simulink model "PowertrainBestFuelController"  (R2019b)
settings: Solver=ode4  StartTime=0.0  StopTime=inf  FixedStep=.01  RelTol=1e-3  EnableMultiTasking=on
model workspace (MAT data in the model file):
  DCT_Param.Transmission.Ratios = [3.78 2.18 1.43 1.03 0.935 0.84]
  DCT_Param.Transmission.Shaft_Inertia_Odd = 0.0023
  DCT_Param.Transmission.Shaft_Inertia_Even = 0.0009
  DCT_Param.Transmission.Shaft_Inertia_Output = 0.008
  DCT_Param.Transmission.Gear_Inertia = 0.001
  DCT_Param.Transmission.Gear_Efficiency = 0.94
  DCT_Param.Transmission.Gear_Ang_Vel_Thr = 0.01
  DCT_Param.Transmission.Shaft_Velocity_Odd = 0
  DCT_Param.Transmission.Shaft_Velocity_Even = 0
  DCT_Param.Transmission.Shaft_Velocity_Output = 0
  DCT_Param.Transmission.Gear_Initial_Velocity = 0
  DCT_Param.Transmission.Abstract.Compliance = 100000
  DCT_Param.Transmission.Abstract.Damping = 10000
  DCT_Param.Transmission.Abstract.Ratio_Time_Const = 0.05
  DCT_Param.Transmission.Abstract.Shift_Gear_Delay = 25
  DCT_Param.Clutch.Torque_Radius = 130
  DCT_Param.Clutch.Num_Friction_Surfaces = 4
  DCT_Param.Clutch.Engagement_Piston_Area = 0.001
  DCT_Param.Clutch.Kinetic_Friction_Coeff = 0.3
  DCT_Param.Clutch.Static_Friction_Coeff = 0.31
  DCT_Param.Clutch.Derating_Factor = 1
  DCT_Param.Clutch.Clutch_Velocity_Tolerance = 0.001
  DCT_Param.Clutch.Threshold_Pressure = 1
  DCT_Param.Clutch.Drag_Torque_Coeff = 0
  DCT_Param.Dog_Clutch.Max_Torque = 1000
  DCT_Param.Dog_Clutch.Teeth_Mean_Radius = 50
  DCT_Param.Dog_Clutch.Tooth_Height = 10
  DCT_Param.Dog_Clutch.Ring_Hub_Clearance = 3
  DCT_Param.Dog_Clutch.Ring_Stop_Stiffness = 1000000
  DCT_Param.Dog_Clutch.Ring_Stop_Damping = 1000
  DCT_Param.Dog_Clutch.Shift_Linkage_Damping = 100
  DCT_Param.Dog_Clutch.Max_Engage_Velocity = 1000000
  DCT_Param.Dog_Clutch.Tooth_Engage_Overlap = 3
  DCT_Param.Vehicle.Mass = 1600
  DCT_Param.Vehicle.Wheels_Per_Axle = 2
  DCT_Param.Vehicle.Distance_CG_FrontAxle = 1.7
  DCT_Param.Vehicle.Distance_CG_RearAxle = 2
  DCT_Param.Vehicle.Distance_CG_Ground = 0.5
  DCT_Param.Vehicle.Frontal_Area = 3
  DCT_Param.Vehicle.Aero_Drag_Coeff = 0.4
  DCT_Param.Vehicle.Initial_Velocity = 0
  DCT_Param.Vehicle.Final_Drive_Ratio = 3.7
  DCT_Param.Vehicle.Final_Drive_Efficiency = 0.86
  DCT_Param.Vehicle.Final_Drive_Vel_Thresh = 0.01
  DCT_Param.Vehicle.Side_Shaft_Inertia = 0.01
  DCT_Param.Vehicle.Side_Shaft_Initial_Velocity = 0
  DCT_Param.Vehicle.Tire.Radius = 0.312
  DCT_Param.Vehicle.Tire.Inertia = 0.5
  DCT_Param.Vehicle.Tire.Initial_Velocity = 0
  DCT_Param.Vehicle.Tire.Slip_Vel_Thresh = 0.1
  DCT_Param.Vehicle.Tire.Nominal_Vertical_Load = 4000
  DCT_Param.Vehicle.Tire.C_Coeff = 1.685
  DCT_Param.Vehicle.Tire.D_Coeff = [1.21 -0.037]
  DCT_Param.Vehicle.Tire.E_Coeff = [0.344 0.095 -0.02 0]
  DCT_Param.Vehicle.Tire.BCD_Coeff = [21.51 -0.163 0.245]
  DCT_Param.Vehicle.Tire.H_Coeff = [-0.002 0.002]
  DCT_Param.Vehicle.Tire.V_Coeff = [0 0]
  DCT_Param.ICE.Max_Power = 100000
  DCT_Param.ICE.Speed_At_Max_Power = 5500
  DCT_Param.ICE.Max_Speed = 7000
  DCT_Param.ICE.Stall_Speed = 200
  DCT_Param.ICE.Shaft_Inertia = 0.2
  DCT_Param.ICE.Initial_Velocity = 800
  DCT_Param.ICE.Idle_Ref_Spd = 800
  DCT_Param.ICE.Engine_Time_Constant = 0.2
  DCT_Param.ICE.Initial_Normalized_Throttle = 0
  DCT_Param.ICE.Speed_Threshold = 20
  DCT_Param.ICE.FC.Speed_Vector = [0 368.421052632 736.842105263 1105.26315789 1473.68421053 1842.10526316 2210.52631579 2578.94736842 2947.36842105 3315.78947368 3684.21052632 4052.63157895 4421.05263158 4789.47368421 5157.89473684 5526.31578947 5894.73684211 6263.15789474 6631.57894737 7000]
  DCT_Param.ICE.FC.Torque_Vector = [0 10.5263157895 21.0526315789 31.5789473684 42.1052631579 52.6315789474 63.1578947368 73.6842105263 84.2105263158 94.7368421053 105.263157895 115.789473684 126.315789474 136.842105263 147.368421053 157.894736842 168.421052632 178.947368421 189.473684211 200]
  DCT_Param.ICE.FC.Consumption_Table = [0.262945178015 0.225304787522 0.201465019624 0.191425874321 0.195187351614 0.212749451502 0.244112173984 0.289275519063 0.348239486736 0.421004077004 0.507569289868 0.607935125326 ... (400 elements, 20x20)]
  DCT_Param.Shift_Map_Example.Pedal_Positions = [0.1 0.4 0.5 0.9]
  DCT_Param.Shift_Map_Example.Upshift_Speeds = [11  20  26  34.5  43; 14  26  35  44.5  55; 17  31  42  52.5  65; 21  39  52  66.5  80]
  DCT_Param.Shift_Map_Example.Downshift_Speeds = [8.9  17  23.6  32.4  40.8; 11.5  22.7  32  41.6  52.2; 14  27  38.1  50  62; 18  33  48  62.6  76.2]
  DCT_Param.Shift_Map_ORIG.Pedal_Positions = [0.1 0.4 0.5 0.9]
  DCT_Param.Shift_Map_ORIG.Upshift_Speeds = [11.5  23.5  35.5  45.5  55.5; 14.5  26.5  38.5  48.5  58.5; 17.5  29.5  41.5  51.5  61.5; 20.5  32.5  44.5  54.5  64.5]
  DCT_Param.Shift_Map_ORIG.Downshift_Speeds = [8.5  20.5  32.5  42.5  52.5; 11.5  23.5  35.5  45.5  55.5; 14.5  26.5  38.5  48.5  58.5; 17.5  29.5  41.5  51.5  61.5]
  DCT_Param.Shift_Map_OPT.Pedal_Positions = [0.1 0.4 0.5 0.9]
  DCT_Param.Shift_Map_OPT.Upshift_Speeds = [17.8469  29.8469  35.8159  41.2981  46.3004; 19.2469  33.9778  43.9778  53.9778  63.9778; 24.5469  41.9778  62.1778  78.5778  106.9778; 27.5469  59.3778  99.0445  109.0445  119.0445]
  DCT_Param.Shift_Map_OPT.Downshift_Speeds = [14.8469  26.8469  32.8159  38.2981  43.3004; 16.2469  30.9778  40.9778  50.9778  60.9778; 21.5469  38.9778  59.1778  75.5778  103.9778; 24.5469  56.3778  96.0445  106.0445  116.0445]
  DCT_Param.Shift_Map.Pedal_Positions = [0.1 0.4 0.5 0.9]
  DCT_Param.Shift_Map.Upshift_Speeds = [11.5  23.5  35.5  45.5  55.5; 14.5  26.5  38.5  48.5  58.5; 17.5  29.5  41.5  51.5  61.5; 20.5  32.5  44.5  54.5  64.5]
  DCT_Param.Shift_Map.Downshift_Speeds = [8.5  20.5  32.5  42.5  52.5; 11.5  23.5  35.5  45.5  55.5; 14.5  26.5  38.5  48.5  58.5; 17.5  29.5  41.5  51.5  61.5]
  DCT_Param.Control.Clutch.Min_Lock_Pressure = 2000000
  DCT_Param.Control.Clutch.Max_Lock_Pressure = 5000000
  DCT_Param.Control.Clutch.Max_Unlock_Pressure = 500000
  DCT_Param.Control.Engine_Start_RPM = 800
  DCT_Param.Control.Engine_Stop_RPM = 790
  DCT_Param.Control.Mode_Logic_TS = 0.1
  DCT_Param.Control.ICE.Kp = 0.02
  DCT_Param.Control.ICE.Ki = 0.01
  DCT_Param.Control.Gen.Kp = 10
  DCT_Param.Control.Gen.Ki = 3
  DCT_Param.Control.Mot.Kp = 500
  DCT_Param.Control.Mot.Ki = 300
  DCT_Param.Control.Veh_Spd.Kp = 0.02
  DCT_Param.Control.Veh_Spd.Ki = 0.04
  DCT_Param.Driver.Kp = 400
  DCT_Param.Driver.Ki = 0.001
  DCT_Param.Driver.Pedal_Filter_Const = 0.01
  DCT_Param.Dog_Clutches.Pulse_Delay = 50
  DCT_Param.Dog_Clutches.Pulse_Length = 20
  DCT_Param.Animation.Teeth_Ratios = [0.338461538462 0.555555555556 0.916666666667 0.96 1.17948717949 1.92307692308]
  DCT_Param.Animation.Teeth_Ratios_Reverse = [0.458333333333 0.75]
  DCT_Param.Shift_Map_OPT506.Pedal_Positions = [0.1 0.4 0.5 0.9]
  DCT_Param.Shift_Map_OPT506.Upshift_Speeds = [18  30.2  48.3  67.3322  77.3429; 20.1  36.85  66.6178  76.7537  86.7537; 21.1  40.25  71.0189  81.0189  91.7873; 24.1  63.75  80.7523  105.9489  115.9489]
  DCT_Param.Shift_Map_OPT506.Downshift_Speeds = [15  27.2  45.3  64.3322  74.3429; 17.1  33.85  63.6178  73.7537  83.7537; 18.1  37.25  68.0189  78.0189  88.7873; 21.1  60.75  77.7523  102.9489  112.9489]
  DCT_Param.Shift_Map_OPTAbsRea176.Pedal_Positions = [0.1 0.4 0.5 0.9]
  DCT_Param.Shift_Map_OPTAbsRea176.Upshift_Speeds = [17.8469  29.8469  35.7875  44.0901  49.4243; 18.9219  34.1312  45.8256  59.7585  69.7585; 32.1719  43.4585  53.51  103.2151  114.6401; 35.1719  59.2585  99.5217  109.5217  119.5217]
  DCT_Param.Shift_Map_OPTAbsRea176.Downshift_Speeds = [14.8469  26.8469  32.7875  41.0901  46.4243; 15.9219  31.1312  42.8256  56.7585  66.7585; 29.1719  40.4585  50.51  100.2151  111.6401; 32.1719  56.2585  96.5217  106.5217  116.5217]
  Downshift_Speeds = [9.5625  23.0625  36.5625  47.8125  59.0625  68.90625  78.75; 12.9375  26.4375  39.9375  51.1875  62.4375  72.84375  83.25; 16.3125  29.8125  43.3125  54.5625  65.8125  76.78125  87.75; 19.6875  33.1875  46.6875  57.9375  69.1875  80.71875  92.25]
  Pedal_Positions = [0.1 0.4 0.5 0.9]
  Upshift_Speeds = [12.9375  26.4375  39.9375  51.1875  62.4375  72.84375  83.25; 16.3125  29.8125  43.3125  54.5625  65.8125  76.78125  87.75; 19.6875  33.1875  46.6875  57.9375  69.1875  80.71875  92.25; 33  52.5  77.25  100.5  138.75  161.875  185]
settings Model: ModifiedByFormat=The MathWorks, Inc.  Creator=The MathWorks, Inc.  LastModifiedBy=The MathWorks, Inc.
settings DataIOCC: SaveFormat=StructureWithTime  DSMLogging=off  ReturnWorkspaceOutputs=off
settings DebuggingCC: ArithmeticOperatorsInVariantConditions=warning
settings SFSimCC: SimUseLocalCustomCode=off  CustomCodeUndefinedFunction=UseInterfaceOnly
settings RTWCC: RTWUseLocalCustomCode=off
settings CodeAppCC: StateflowObjectComments=on
settings GRTTargetCC: TargetLangStandard=C89/C90 (ANSI)
settings ConfigComp: CovMetricSettings=dsw  CovHtmlReporting=on  CovSaveCumulativeToWorkspaceVar=on  CovSaveSingleToWorkspaceVar=on  CovShowResultsExplorer=off  CovExternalEMLEnable=off

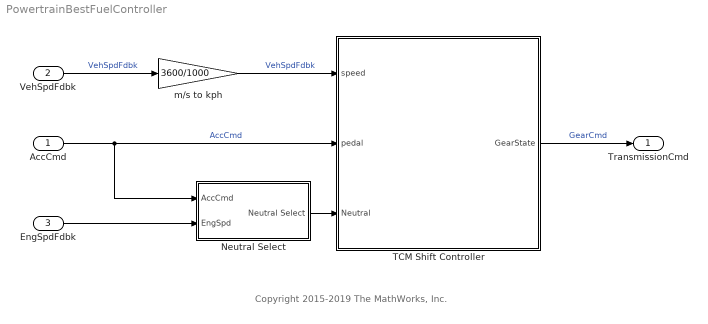
== system PowertrainBestFuelController ==
  note: Copyright 2015-2019 The MathWorks, Inc.
  AccCmd : Inport
  VehSpdFdbk : Inport  Port=2
  EngSpdFdbk : Inport  Port=3
  Neutral Select : Subsystem
  TCM Shift Controller : Stateflow chart  TreatAsAtomicUnit=on
  m/s to kph : Gain  Gain=3600/1000
  TransmissionCmd : Outport  VectorParamsAs1DForOutWhenUnconnected=off
  wires:
  AccCmd/1 -> Neutral Select/1(AccCmd), TCM Shift Controller/2(pedal)  "AccCmd"
  m/s to kph/1 -> TCM Shift Controller/1(speed)  "VehSpdFdbk"
  VehSpdFdbk/1 -> m/s to kph/1  "VehSpdFdbk"
  EngSpdFdbk/1 -> Neutral Select/2(EngSpd)
  Neutral Select/1(Neutral Select) -> TCM Shift Controller/3(Neutral)
  TCM Shift Controller/1(GearState) -> TransmissionCmd/1  "GearCmd"

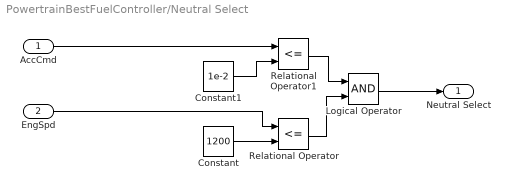
== system PowertrainBestFuelController/Neutral Select ==
  AccCmd : Inport
  EngSpd : Inport  Port=2
  Constant : Constant  Value=1200
  Constant1 : Constant  Value=1e-2
  Logical Operator : Logic  AllPortsSameDT=off  OutDataTypeStr=boolean
  Relational Operator : RelationalOperator  Operator=<=  OutDataTypeStr=boolean  RndMeth=Simplest
  Relational Operator1 : RelationalOperator  Operator=<=  OutDataTypeStr=boolean  RndMeth=Simplest
  Neutral Select : Outport  VectorParamsAs1DForOutWhenUnconnected=off
  wires:
  EngSpd/1 -> Relational Operator/1
  Relational Operator1/1 -> Logical Operator/1
  AccCmd/1 -> Relational Operator1/1
  Constant1/1 -> Relational Operator1/2
  Logical Operator/1 -> Neutral Select/1
  Constant/1 -> Relational Operator/2
  Relational Operator/1 -> Logical Operator/2

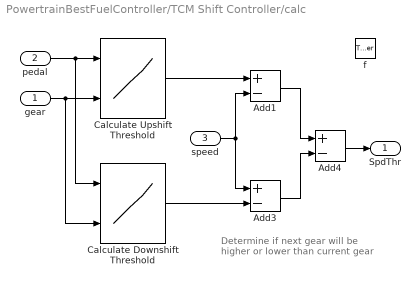
== system PowertrainBestFuelController/TCM Shift Controller/calc ==
  note: Determine if next gear will be
      | higher or lower than current gear
  gear : Inport
  pedal : Inport  Port=2
  speed : Inport  Port=3
  f : TriggerPort  TriggerType=function-call  VariantControl=Variant  StatesWhenEnabling=reset
      settings: CopyFcn=Stateflow.SLINSF.SimulinkMan.removeBlockPreDeleteFcn  PreDeleteFcn=Stateflow.SLINSF.SimulinkMan.unsafePredeleteFcn
  Add1 : Sum  Inputs=+-
  Add3 : Sum  Inputs=+-
  Add4 : Sum  Inputs=+-
  Calculate Upshift Threshold : Lookup_n-D  BreakpointsForDimension1=Pedal_Positions  BreakpointsForDimension2=1:7  Table=Upshift_Speeds  ExtrapMethod=Clip  UseLastTableValue=on  InternalRulePriority=Speed  RndMeth=Simplest  InputSameDT=on
  Calculate Downshift Threshold : Lookup_n-D  BreakpointsForDimension1=Pedal_Positions  BreakpointsForDimension2=2:8  Table=Downshift_Speeds  ExtrapMethod=Clip  UseLastTableValue=on  InternalRulePriority=Speed  RndMeth=Simplest  InputSameDT=on
  SpdThr : Outport  VectorParamsAs1DForOutWhenUnconnected=off
  wires:
  pedal/1 -> Calculate Downshift Threshold/1, Calculate Upshift Threshold/1
  gear/1 -> Calculate Downshift Threshold/2, Calculate Upshift Threshold/2
  Calculate Downshift Threshold/1 -> Add3/2
  Calculate Upshift Threshold/1 -> Add1/1
  speed/1 -> Add1/2, Add3/1
  Add1/1 -> Add4/1
  Add3/1 -> Add4/2
  Add4/1 -> SpdThr/1

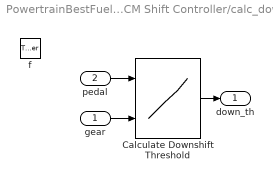
== system PowertrainBestFuelController/TCM Shift Controller/calc_down ==
  gear : Inport
  pedal : Inport  Port=2
  f : TriggerPort  TriggerType=function-call  VariantControl=Variant  StatesWhenEnabling=reset
      settings: CopyFcn=Stateflow.SLINSF.SimulinkMan.removeBlockPreDeleteFcn  PreDeleteFcn=Stateflow.SLINSF.SimulinkMan.unsafePredeleteFcn
  Calculate Downshift Threshold : Lookup_n-D  BreakpointsForDimension1=Pedal_Positions  BreakpointsForDimension2=2:8  Table=Downshift_Speeds  ExtrapMethod=Clip  UseLastTableValue=on  InternalRulePriority=Speed  RndMeth=Simplest  InputSameDT=on
  down_th : Outport  VectorParamsAs1DForOutWhenUnconnected=off
  wires:
  Calculate Downshift Threshold/1 -> down_th/1
  gear/1 -> Calculate Downshift Threshold/2
  pedal/1 -> Calculate Downshift Threshold/1

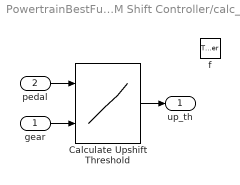
== system PowertrainBestFuelController/TCM Shift Controller/calc_up ==
  gear : Inport
  pedal : Inport  Port=2
  f : TriggerPort  TriggerType=function-call  VariantControl=Variant  StatesWhenEnabling=reset
      settings: CopyFcn=Stateflow.SLINSF.SimulinkMan.removeBlockPreDeleteFcn  PreDeleteFcn=Stateflow.SLINSF.SimulinkMan.unsafePredeleteFcn
  Calculate Upshift Threshold : Lookup_n-D  BreakpointsForDimension1=Pedal_Positions  BreakpointsForDimension2=1:7  Table=Upshift_Speeds  ExtrapMethod=Clip  UseLastTableValue=on  InternalRulePriority=Speed  RndMeth=Simplest  InputSameDT=on
  up_th : Outport  VectorParamsAs1DForOutWhenUnconnected=off
  wires:
  Calculate Upshift Threshold/1 -> up_th/1
  pedal/1 -> Calculate Upshift Threshold/1
  gear/1 -> Calculate Upshift Threshold/2

== stateflow chart PowertrainBestFuelController/TCM Shift Controller ==
  settings: sampleTime=0.01
  state GearState [parallel]
    settings: executionOrder=1
    state Neutral
      en:
      GearState = 0;
    state G1
      en:
      GearState = 1;
    state G2
      en:
      GearState = 2;
      du:
      [SpdThr] = calc(2,pedal,speed);
    state G3
      en:
      GearState = 3;
      du:
      [SpdThr] = calc(3,pedal,speed);
    state G8
      en:
      GearState = 8;
    state G7
      en:
      GearState = 7;
    state G6
      en:
      GearState = 6;
    state G5
      en:GearState=5;
      du:[SpdThr]=calc(5,pedal,speed);
    state G4
      en:
      GearState = 4;
      du:
      [SpdThr] = calc(4,pedal,speed);
    (default) -> G1
    Neutral -> G1 : [~Neutral]
    G1 -> G2 [order 1] : Up
    G2 -> G3 [order 1] : Up
    G1 -> Neutral [order 2] : [Neutral]
    G2 -> G1 [order 2] : Down
    G3 -> G2 [order 2] : Down
    G3 -> G4 [order 1] : Up
    G4 -> G3 [order 2] : Down
    G7 -> G8 [order 1] : Up
    G5 -> G6 [order 1] : Up
    G6 -> G7 [order 1] : Up
    G4 -> G5 [order 1] : Up
    G5 -> G4 [order 2] : Down
    G6 -> G5 [order 2] : Down
    G7 -> G6 [order 2] : Down
    G8 -> G7 : Down
  state SelectionState [parallel]
    du:[up_th]=calc_up(GearState,pedal);
    du:[down_th]=calc_down(GearState,pedal);
    settings: executionOrder=2
    state SteadyState
      en:
      clutchControl = 0;
    state preDownShifting
    state preUpShifting
    state UpShifting
      en:
      GearState = GearState + 0.5;
    state DownShifting
      en:
      GearState = GearState - 0.5;
    (default) -> SteadyState
    SteadyState -> (junction 62) [order 1] : [speed < down_th && ...
        | GearState >1]
    SteadyState -> (junction 128) [order 2] : [speed > up_th &&...
        | GearState <= 5 && ...
        | floor(GearState) == GearState]
    (junction 62) -> preDownShifting
    (junction 128) -> preUpShifting
    (junction 168) -> SteadyState
    (junction 23) -> SteadyState
    (junction 161) -> SteadyState
    preDownShifting -> (junction 168) [order 2] : [speed >= down_th]
    preUpShifting -> (junction 161) [order 2] : [speed <= up_th]
    preUpShifting -> UpShifting [order 1] : after(0.5,sec)
        | [speed>up_th]
    preDownShifting -> DownShifting [order 1] : after(0.5, sec)
        | [speed < down_th - 2]
    DownShifting -> (junction 23) : {GearState.Down;}
    UpShifting -> (junction 23) : {GearState.Up;}
  state up_th = calc_up(gear,pedal) [function]
  state down_th = calc_down(gear,pedal) [function]
  state SpdThr = calc(gear,pedal,speed) [function]
  data: gear function_input; pedal function_input; up_th function_output; gear function_input; pedal function_input; down_th function_output; gear function_input; pedal function_input; SpdThr function_output; speed function_input; GearState output double; speed input; pedal input; clutchControl local double; SpdThr local double; Neutral input; up_th local double; down_th local double
  events: Up local EITHER_EDGE_EVENT; Down local EITHER_EDGE_EVENT
